simulink model "pidcontrollerdesign"  (R2023a)
settings: Solver=VariableStepAuto  StartTime=0.0  StopTime=20  RelTol=1e-3
libraries: spspowerguiLib x1
settings Model: Creator=GYANESH  LastModifiedBy=GYANESH

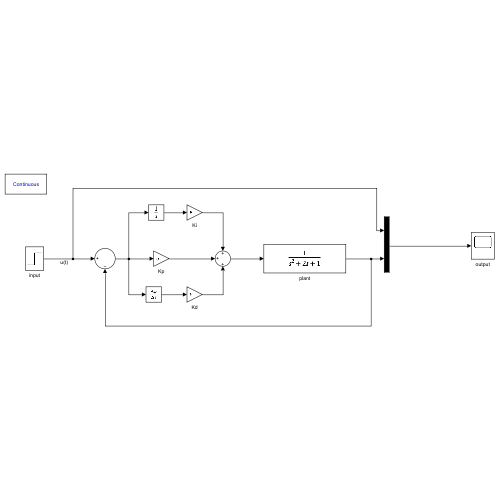
[thumbnail: Simulink's stored preview of the top-level diagram]
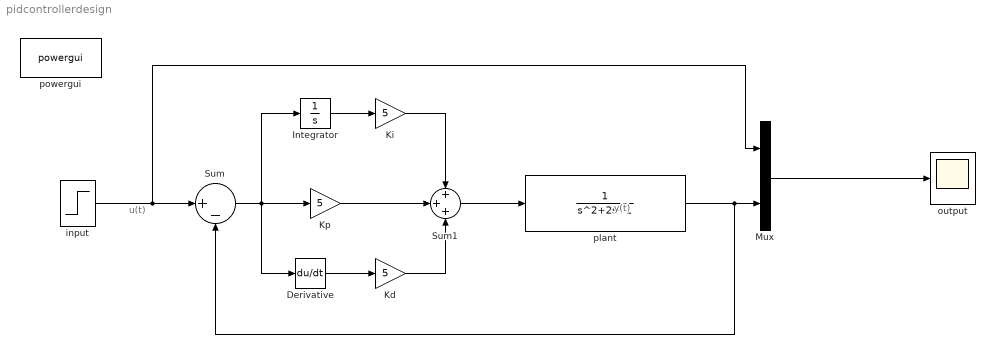
== system pidcontrollerdesign ==
  note: y(t)
  note: u(t)
  Derivative : Derivative
  Integrator : Integrator
  Kd : Gain  Gain=5
  Ki : Gain  Gain=5
  Kp : Gain  Gain=5
  Mux : Mux  Inputs=2
  Sum : Sum  Inputs=|+-
  Sum1 : Sum  Inputs=+++
  input : Step  SampleTime=0
  output : Scope
  plant : TransferFcn  Denominator=[1,2,1]
  powergui : spspowerguiLib/powergui  Priority=1  SimulationMode=Continuous  SampleTime=50e-6  frequency=60  Iterations=50  frequencyindice=60  Pbase=100e6  ErrMax=1e-4  UnitsV=kV  UnitsW=MW  buscounter=0  FunctionMessages=off  echomessages=off  EnableUseOfTLC=off  CurrentSourceSwitches=off  DisableSnubberDevices=off  DisableRonSwitches=off  DisableVfSwitches=off  DisplayEquations=off  AutomaticDiscreteSolvers=off  SolverType=Tustin/Backward Euler (TBE)  Interpol=off  ExternalGateDelay=off  methode=off  Ts=100  x0status=blocks  SPID=on  SwTol=0  HookPort=off  NonlinearTolerance=1e-4  nMaxIteration=100  ContinueOnMaxIteration=off  RestoreLinks=warning  ResistiveCurrentMeasurement=off  Frange=[0:2:500]  Ylog=off  Xlog=on  ShowGrid=off  save=off  variable=ZData  structure=0  ZoomFFT=off  StartTime=0.0  cycles=1  DisplayStyle=1  fundamental=60  FreqAxis=off  MaxFrequency=1000  frequencyindicesteady=1  RmsSteady=1  display=off
  wires:
  input/1 -> Mux/1, Sum/1
  plant/1 -> Sum/2, Mux/2
  Mux/1 -> output/1
  Integrator/1 -> Ki/1
  Derivative/1 -> Kd/1
  Sum/1 -> Derivative/1, Integrator/1, Kp/1
  Kp/1 -> Sum1/2
  Sum1/1 -> plant/1
  Ki/1 -> Sum1/1
  Kd/1 -> Sum1/3
